simulink model "Cascade_ACC_Para"  (R2020b)
settings: Solver=FixedStepAuto  StartTime=0.0  StopTime=1830  FixedStep=0.02  RelTol=1e-3
model workspace (MAT data in the model file):
  P_a_x = [-10 0 10]
  P_a_y = [-7 0 7]
  P_v_x = [-100 0 100]
  P_v_y = [-7 0 7]
  Range_Sensor = 200
  a_max_x = [0 5 20 50]
  a_max_y = [4 4 2 2]
  a_min_x = [-1 0 0.0001 5 20 50]
  a_min_y = [0 0 -5 -5 -3.5 -3.5]
  cycle_t = [0 1 2 3 4 5 6 7 8 9 10 11 ... (1083 elements, 1083x1)]
  cycle_v = [0 0 0 0 0 0 2 9.4 16.3 19.7 21.2 24.1 ... (1083 elements, 1083x1)]
  d0 = 4
  j_min_x = [0 5 20 50]
  j_min_y = [-5 -5 -2.5 -2.5]
  speed_set = 120
  t_sensor = 0.2
  t_set = 2
libraries: simulink x4, SignalEditorBlockLib x1
settings Model: OrderedModelArguments=off  Creator=duanx  LastModifiedBy=duanx

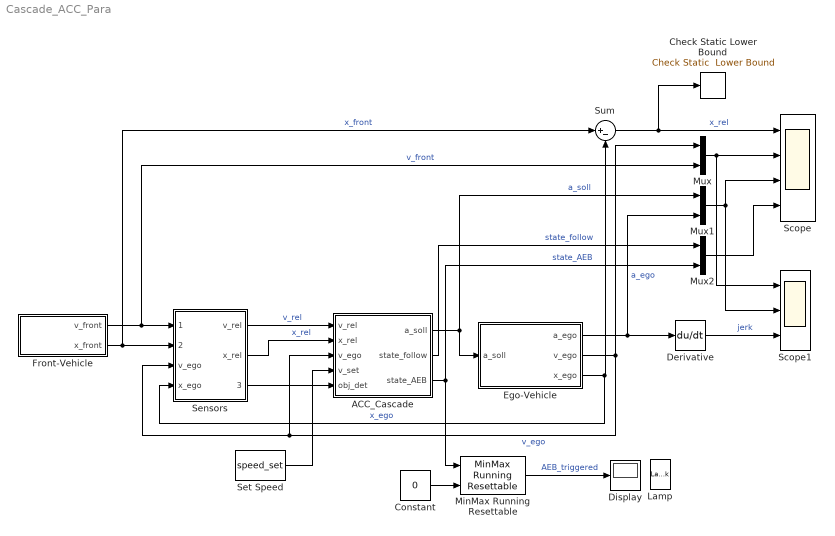
== system Cascade_ACC_Para ==
  ACC_Cascade : Subsystem
  Check Static Lower Bound : simulink/Model Verification/Check Static  Lower Bound  Description=0 <= u  min=0  min_included=on  enabled=on  stopWhenAssertionFail=on  export=off  icon=graphic
  Constant : Constant  Value=0
  Derivative : Derivative
  Display : Display
  Ego-Vehicle : Subsystem
  Front-Vehicle : Subsystem
  Lamp : LampBlock
  MinMax Running Resettable : simulink/Math Operations/MinMax Running Resettable  Function=max  vinit=0.0
  Mux : Mux  Inputs=2
  Mux1 : Mux  Inputs=2
  Mux2 : Mux  Inputs=2
  Scope : Scope  NumInputPorts=4
  Scope1 : Scope  NumInputPorts=3
  Sensors : Subsystem
  Set Speed : Constant  Value=speed_set
  Sum : Sum  Inputs=|+-
  wires:
  Front-Vehicle/1(v_front) -> Mux/2, Sensors/1(v_front)  "v_front"
  Front-Vehicle/2(x_front) -> Sensors/2(x_front), Sum/1  "x_front"
  Ego-Vehicle/2(v_ego) -> ACC_Cascade/3(v_ego), Sensors/3(v_ego), Mux/1  "v_ego"
  Ego-Vehicle/3(x_ego) -> Sensors/4(x_ego), Sum/2  "x_ego"
  Sensors/1(v_rel) -> ACC_Cascade/1(v_rel)  "v_rel"
  Sensors/2(x_rel) -> ACC_Cascade/2(x_rel)  "x_rel"
  ACC_Cascade/1(a_soll) -> Ego-Vehicle/1(a_soll), Mux1/1  "a_soll"
  Mux/1 -> Scope1/1, Scope/2
  Ego-Vehicle/1(a_ego) -> Mux1/2, Derivative/1  "a_ego"
  Mux1/1 -> Scope/3, Scope1/2
  Sensors/3(Obj_det) -> ACC_Cascade/5(obj_det)
  Set Speed/1 -> ACC_Cascade/4(v_set)
  Derivative/1 -> Scope1/3  "jerk"
  ACC_Cascade/3(state_AEB) -> Mux2/2, MinMax Running Resettable/1  "state_AEB"
  MinMax Running Resettable/1 -> Display/1  "AEB_triggered"
  Mux2/1 -> Scope/4
  ACC_Cascade/2(state_follow) -> Mux2/1  "state_follow"
  Sum/1 -> Check Static Lower Bound/1, Scope/1  "x_rel"
  Constant/1 -> MinMax Running Resettable/2

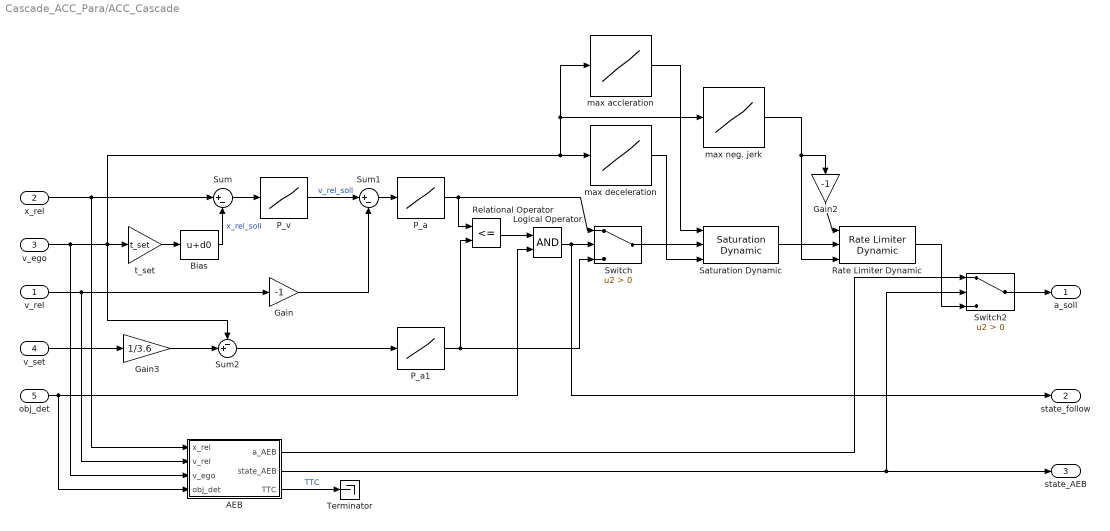
== system Cascade_ACC_Para/ACC_Cascade ==
  v_rel : Inport  Unit=m/s
  x_rel : Inport  Port=2  Unit=m
  v_ego : Inport  Port=3  Unit=m/s
  v_set : Inport  Port=4  Unit=km/h
  obj_det : Inport  Port=5
  AEB : Subsystem
  Bias : Bias  Bias=d0
  Gain : Gain  Gain=-1
  Gain2 : Gain  Gain=-1
  Gain3 : Gain  Gain=1/3.6
  Logical Operator : Logic  AllPortsSameDT=off  OutDataTypeStr=boolean
  P_a : Lookup_n-D  NumberOfTableDimensions=1  BreakpointsForDimension1=P_a_x  Table=P_a_y  InternalRulePriority=Speed  RndMeth=Simplest  InputSameDT=on
  P_a1 : Lookup_n-D  NumberOfTableDimensions=1  BreakpointsForDimension1=P_a_x  Table=P_a_y  InternalRulePriority=Speed  RndMeth=Simplest  InputSameDT=on
  P_v : Lookup_n-D  NumberOfTableDimensions=1  BreakpointsForDimension1=P_v_x  Table=P_v_y  InternalRulePriority=Speed  RndMeth=Simplest  InputSameDT=on
  Rate Limiter Dynamic : simulink/Discontinuities/Rate Limiter Dynamic
  Relational Operator : RelationalOperator  Operator=<=  OutDataTypeStr=boolean  RndMeth=Simplest
  Saturation Dynamic : simulink/Discontinuities/Saturation Dynamic  OutMin=[]  OutMax=[]  OutDataTypeStr=Inherit: Same as second input  OutDataType=fixdt(1, 16)  OutScaling=2^-10  DoSatur=off
  Sum : Sum  Inputs=|+-
  Sum1 : Sum  Inputs=|+-
  Sum2 : Sum  Inputs=-+|
  Switch : Switch  Criteria=u2 > Threshold
  Switch2 : Switch  Criteria=u2 > Threshold
  Terminator : Terminator
  max accleration : Lookup_n-D  NumberOfTableDimensions=1  BreakpointsForDimension1=a_max_x  Table=a_max_y  InternalRulePriority=Speed  RndMeth=Simplest  InputSameDT=on
  max deceleration : Lookup_n-D  NumberOfTableDimensions=1  BreakpointsForDimension1=a_min_x  Table=a_min_y  InternalRulePriority=Speed  RndMeth=Simplest  InputSameDT=on
  max neg. jerk : Lookup_n-D  NumberOfTableDimensions=1  BreakpointsForDimension1=j_min_x  Table=j_min_y  InternalRulePriority=Speed  RndMeth=Simplest  InputSameDT=on
  t_set : Gain  Gain=t_set
  a_soll : Outport
  state_follow : Outport  Port=2
  state_AEB : Outport  Port=3
  wires:
  Sum/1 -> P_v/1
  x_rel/1 -> AEB/1(x_rel), Sum/1
  t_set/1 -> Bias/1
  Sum1/1 -> P_a/1
  P_v/1 -> Sum1/1  "v_rel_soll"
  v_rel/1 -> AEB/2(v_rel), Gain/1
  Gain/1 -> Sum1/2
  P_a/1 -> Relational Operator/1, Switch/1
  Sum2/1 -> P_a1/1
  P_a1/1 -> Switch/3, Relational Operator/2
  Logical Operator/1 -> state_follow/1, Switch/2
  Relational Operator/1 -> Logical Operator/1
  obj_det/1 -> Logical Operator/2, AEB/4(obj_det)
  Switch/1 -> Saturation Dynamic/2
  Saturation Dynamic/1 -> Rate Limiter Dynamic/2
  max accleration/1 -> Saturation Dynamic/1
  max neg. jerk/1 -> Gain2/1, Rate Limiter Dynamic/3
  Gain2/1 -> Rate Limiter Dynamic/1
  v_set/1 -> Gain3/1
  Gain3/1 -> Sum2/2
  Bias/1 -> Sum/2  "x_rel_soll"
  v_ego/1 -> AEB/3(v_ego), Sum2/1, t_set/1, max accleration/1, max neg. jerk/1, max deceleration/1
  max deceleration/1 -> Saturation Dynamic/3
  Switch2/1 -> a_soll/1
  AEB/2(state_AEB) -> state_AEB/1, Switch2/2
  AEB/1(a_AEB) -> Switch2/1
  Rate Limiter Dynamic/1 -> Switch2/3
  AEB/3(TTC) -> Terminator/1  "TTC"

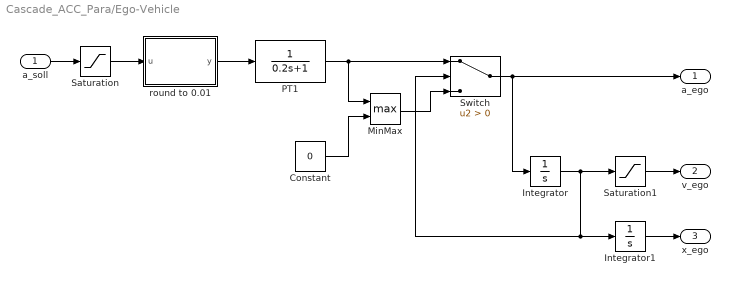
== system Cascade_ACC_Para/Ego-Vehicle ==
  a_soll : Inport
  Constant : Constant  Value=0
  Integrator : Integrator
  Integrator1 : Integrator
  MinMax : MinMax  Function=max  Inputs=2
  PT1 : TransferFcn  Denominator=[0.2 1]
  Saturation : Saturate  UpperLimit=6  LowerLimit=-8
  Saturation1 : Saturate  UpperLimit=100  LowerLimit=0
  Switch : Switch  Criteria=u2 > Threshold
  round to 0.01 : MATLAB Function
  a_ego : Outport
  v_ego : Outport  Port=2
  x_ego : Outport  Port=3
  wires:
  PT1/1 -> Switch/1, MinMax/1
  Integrator/1 -> Integrator1/1, Switch/2, Saturation1/1
  Integrator1/1 -> x_ego/1
  a_soll/1 -> Saturation/1
  Saturation/1 -> round to 0.01/1(u)
  Switch/1 -> Integrator/1, a_ego/1
  MinMax/1 -> Switch/3
  Constant/1 -> MinMax/2
  Saturation1/1 -> v_ego/1
  round to 0.01/1(y) -> PT1/1

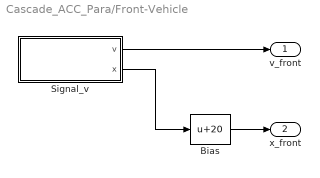
== system Cascade_ACC_Para/Front-Vehicle ==
  Bias : Bias  Bias=20
  Signal_v : Subsystem
  v_front : Outport  Unit=m/s
  x_front : Outport  Port=2  Unit=m
  wires:
  Bias/1 -> x_front/1
  Signal_v/1(v) -> v_front/1
  Signal_v/2(x) -> Bias/1

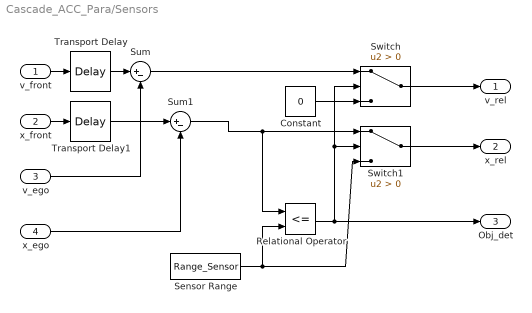
== system Cascade_ACC_Para/Sensors ==
  v_front : Inport  Unit=m/s
  x_front : Inport  Port=2  Unit=m
  v_ego : Inport  Port=3  Unit=m/s
  x_ego : Inport  Port=4  Unit=m
  Constant : Constant  Value=0
  Relational Operator : RelationalOperator  Operator=<=  OutDataTypeStr=boolean  RndMeth=Simplest
  Sensor Range : Constant  Value=Range_Sensor
  Sum : Sum  Inputs=|+-
  Sum1 : Sum  Inputs=|+-
  Switch : Switch  Criteria=u2 > Threshold
  Switch1 : Switch  Criteria=u2 > Threshold
  Transport Delay : TransportDelay  DelayTime=t_sensor
  Transport Delay1 : TransportDelay  DelayTime=t_sensor
  v_rel : Outport
  x_rel : Outport  Port=2
  Obj_det : Outport  Port=3  OutDataTypeStr=boolean
  wires:
  v_ego/1 -> Sum/2
  x_front/1 -> Transport Delay1/1
  x_ego/1 -> Sum1/2
  Sum1/1 -> Switch1/1, Relational Operator/1
  Relational Operator/1 -> Switch1/2, Switch/2, Obj_det/1
  Switch/1 -> v_rel/1
  Switch1/1 -> x_rel/1
  Sum/1 -> Switch/1
  Constant/1 -> Switch/3
  Sensor Range/1 -> Relational Operator/2, Switch1/3
  Transport Delay/1 -> Sum/1
  v_front/1 -> Transport Delay/1
  Transport Delay1/1 -> Sum1/1

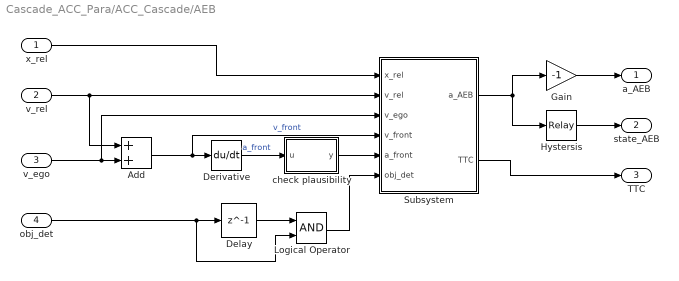
== system Cascade_ACC_Para/ACC_Cascade/AEB ==
  x_rel : Inport
  v_rel : Inport  Port=2
  v_ego : Inport  Port=3
  obj_det : Inport  Port=4
  Add : Sum
  Delay : Delay  DelayLength=1  InitialCondition=0
  Derivative : Derivative
  Gain : Gain  Gain=-1
  Hystersis : Relay  OnSwitchValue=4  OffSwitchValue=0  OutDataTypeStr=Inherit: Inherit via back propagation
  Logical Operator : Logic  AllPortsSameDT=off  OutDataTypeStr=boolean
  Subsystem : Subsystem
  check plausibility : MATLAB Function  TreatAsAtomicUnit=on
  a_AEB : Outport
  state_AEB : Outport  Port=2
  TTC : Outport  Port=3
  wires:
  v_rel/1 -> Add/1, Subsystem/2(v_rel)
  v_ego/1 -> Subsystem/3(v_ego), Add/2
  Add/1 -> Subsystem/4(v_front), Derivative/1  "v_front"
  Hystersis/1 -> state_AEB/1
  obj_det/1 -> Logical Operator/2, Delay/1
  Delay/1 -> Logical Operator/1
  Subsystem/1(a_AEB) -> Gain/1, Hystersis/1
  x_rel/1 -> Subsystem/1(x_rel)
  Gain/1 -> a_AEB/1
  Derivative/1 -> check plausibility/1(u)  "a_front"
  Logical Operator/1 -> Subsystem/6(obj_det)
  check plausibility/1(y) -> Subsystem/5(a_front)
  Subsystem/2(TTC) -> TTC/1

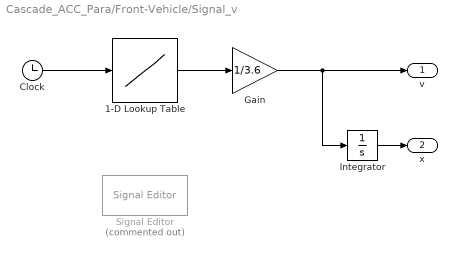
== system Cascade_ACC_Para/Front-Vehicle/Signal_v ==
  1-D Lookup Table : Lookup_n-D  NumberOfTableDimensions=1  BreakpointsForDimension1=cycle_t  Table=cycle_v  InterpMethod=Akima spline  InternalRulePriority=Speed  RndMeth=Simplest  InputSameDT=on
  Clock : Clock
  Gain : Gain  Gain=1/3.6
  Integrator : Integrator
  Signal Editor : SignalEditorBlockLib/Signal Editor  Commented=on  FileName=Signal_v_profile.mat  ActiveScenario=WLTC  ActiveSignal=v  IsBus=off  OutputBusObjectStr=Bus: BusObject  SampleTime=0  ZeroCross=off  OutputAfterFinalValue=Holding final value  Unit=km/h  PreserveSignalName=on
  v : Outport  Unit=m/s
  x : Outport  Port=2  Unit=m
  wires:
  Integrator/1 -> x/1
  Gain/1 -> Integrator/1, v/1
  1-D Lookup Table/1 -> Gain/1
  Clock/1 -> 1-D Lookup Table/1

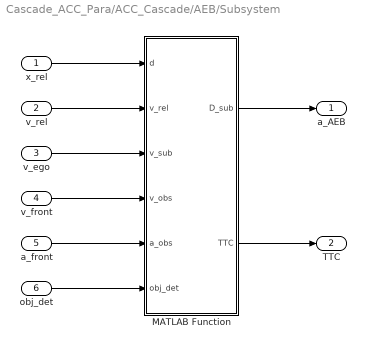
== system Cascade_ACC_Para/ACC_Cascade/AEB/Subsystem ==
  x_rel : Inport
  v_rel : Inport  Port=2
  v_ego : Inport  Port=3
  v_front : Inport  Port=4
  a_front : Inport  Port=5
  obj_det : Inport  Port=6
  MATLAB Function : MATLAB Function  TreatAsAtomicUnit=on
  a_AEB : Outport
  TTC : Outport  Port=2
  wires:
  x_rel/1 -> MATLAB Function/1(d)
  v_rel/1 -> MATLAB Function/2(v_rel)
  v_ego/1 -> MATLAB Function/3(v_sub)
  v_front/1 -> MATLAB Function/4(v_obs)
  a_front/1 -> MATLAB Function/5(a_obs)
  MATLAB Function/1(D_sub) -> a_AEB/1
  obj_det/1 -> MATLAB Function/6(obj_det)
  MATLAB Function/2(TTC) -> TTC/1

== matlab function Cascade_ACC_Para/ACC_Cascade/AEB/check plausibility ==
  data: u input; y output
function y = fcn(u)
if abs(u) < 8
    y = u;
else
    y = 0;
end

== matlab function Cascade_ACC_Para/ACC_Cascade/AEB/Subsystem/MATLAB Function ==
  data: d input; D_sub output; v_rel input; v_sub input; v_obs input; a_obs input; TTC output; obj_det input
function [D_sub,TTC] = fcn(d,v_rel,v_sub,v_obs,a_obs,obj_det)
if obj_det
    % 1 - not approaching
    if v_rel >= 0
        D_sub = 0;
        TTC = inf;
    else
        v_diff = - v_rel;
        d = max(d - 2,0);
        % 2 - front vehicle not decelerating
        TTC = d / v_diff;
        if a_obs >= 0
            D_sub = v_diff ^2 / (2 * d);
        else
            D_obs = - a_obs;        
            D_sub = 0;
            D_rel = D_obs - D_sub;
            % 3 - front vehicle braking
            %TTC = (sqrt(v_diff ^2 + 2 * D_rel * d) - v_diff)/D_rel;
            if v_obs / D_obs > TTC
                D_sub = D_obs + v_diff ^2 / (2 * d);
            else
                % 4 - front vehicle braking to a stop
                %TTC = (v_sub - sqrt(v_sub ^2 - 2 * D_sub * d - v_obs ^2 * D_sub / D_obs)) / D_sub;
                D_sub = v_sub ^2 /(2 * (d + v_obs ^2 / (2 * D_obs)));
            end
        end
    end
else
    D_sub = 0;
    TTC = inf;
end
if v_sub <= 0
    D_sub = 0;
end

== matlab function Cascade_ACC_Para/Ego-Vehicle/round to 0.01 ==
  data: u input; y output
function y = round01(u)
    value = abs(u) * 100;
    sign = u > 0;
    value = floor(value);
    if sign
        y = value / 100;
    else
        y = - value / 100;
    end
end
